simulink model "GaussianDistEstimator"  (R2021b)
settings: Solver=VariableStepAuto  StartTime=0.0  StopTime=10.0  RelTol=1e-3
values from neighbouring files (symbols this model uses):
  nt = 5    [test_disturbance_recursive.m]
  sigma_noise = std_n    (= 0.01)    [test_disturbance_recursive.m]
  tau = [sigma;l]    [test_disturbance_recursive.m]
  tc = 1e-3    (= 0.001)    [test_disturbance_recursive.m]
  v_vbuf = linspace(-1,1,nv)'    [test_disturbance_recursive.m]
libraries: cstblocks x5
settings Model: Creator=manue  LastModifiedBy=manue
settings DataIOCC: ExternalInput=[t, u, v_, n]  LoadExternalInput=on

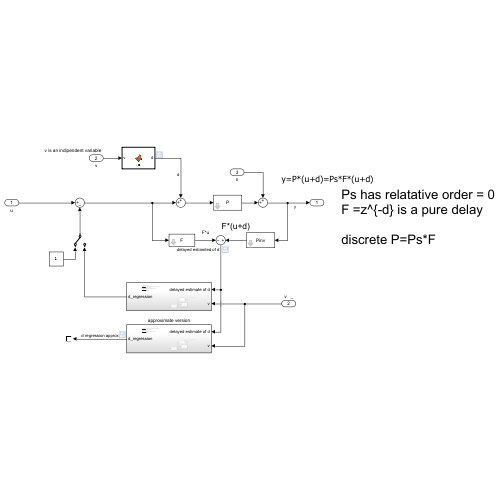
[thumbnail: Simulink's stored preview of the top-level diagram]
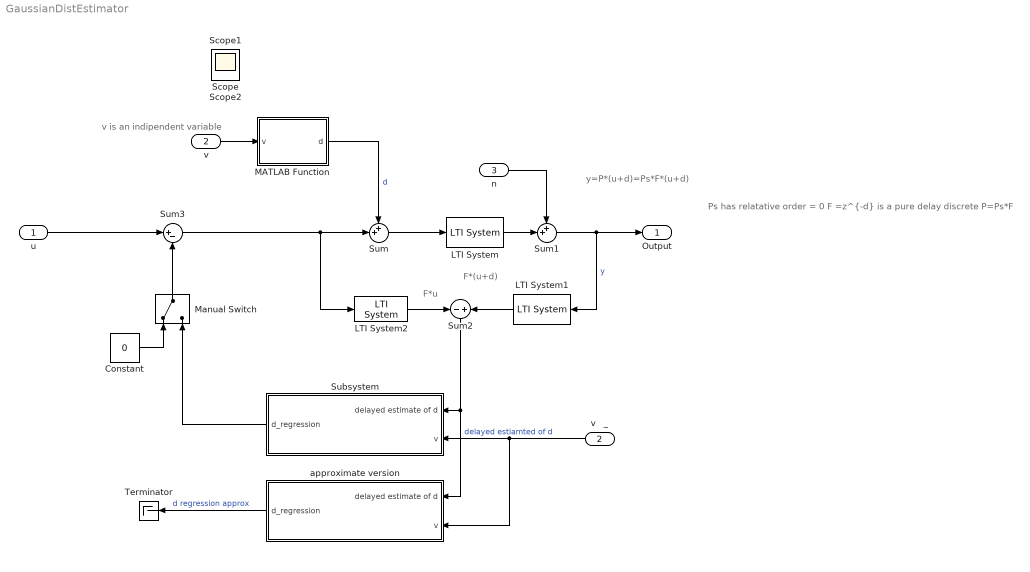
== system GaussianDistEstimator ==
  note: F*u
  note: F*(u+d)
  note: y=P*(u+d)=Ps*F*(u+d)
  note: v is an indipendent variable
  note: Ps has relatative order = 0
      | F =z^{-d} is a pure delay
      |
      | discrete P=Ps*F
  u : Inport
  v : Inport  Port=2
  n : Inport  Port=3
  Constant : Constant  Value=0
  LTI System : cstblocks/LTI System  sys=P  IC=[]
  LTI System1 : cstblocks/LTI System  sys=Pinv  IC=[]
  LTI System2 : cstblocks/LTI System  sys=F  IC=[]
  MATLAB Function : MATLAB Function  TreatAsAtomicUnit=on
  Manual Switch : ManualSwitch
  Subsystem : Subsystem
  Sum : Sum  Inputs=++|
  Sum1 : Sum  Inputs=++|
  Sum2 : Sum  Inputs=-+
  Sum3 : Sum  Inputs=|+-
  Terminator : Terminator
  approximate version : Subsystem
  v   _ : InportShadow  Port=2
  Output : Outport
  Scope : Scope
  Scope1 : Scope
  Scope2 : Scope
  wires:
  Sum/1 -> LTI System/1
  LTI System/1 -> Sum1/2
  Sum3/1 -> LTI System2/1, Sum/2
  Sum1/1 -> LTI System1/1, Output/1  "y"
  v/1 -> MATLAB Function/1(v)
  LTI System2/1 -> Sum2/1
  LTI System1/1 -> Sum2/2
  MATLAB Function/1(d) -> Sum/1  "d"
  u/1 -> Sum3/1
  Manual Switch/1 -> Sum3/2
  Constant/1 -> Manual Switch/1
  n/1 -> Sum1/1
  Sum2/1 -> approximate version/1(delayed estimate of d), Subsystem/1(delayed estimate of d)  "delayed estiamted of d"
  v   _/1 -> approximate version/2(v), Subsystem/2(v)
  Subsystem/1(d_regression) -> Manual Switch/2
  approximate version/1(d_regression) -> Terminator/1  "d regression approx"

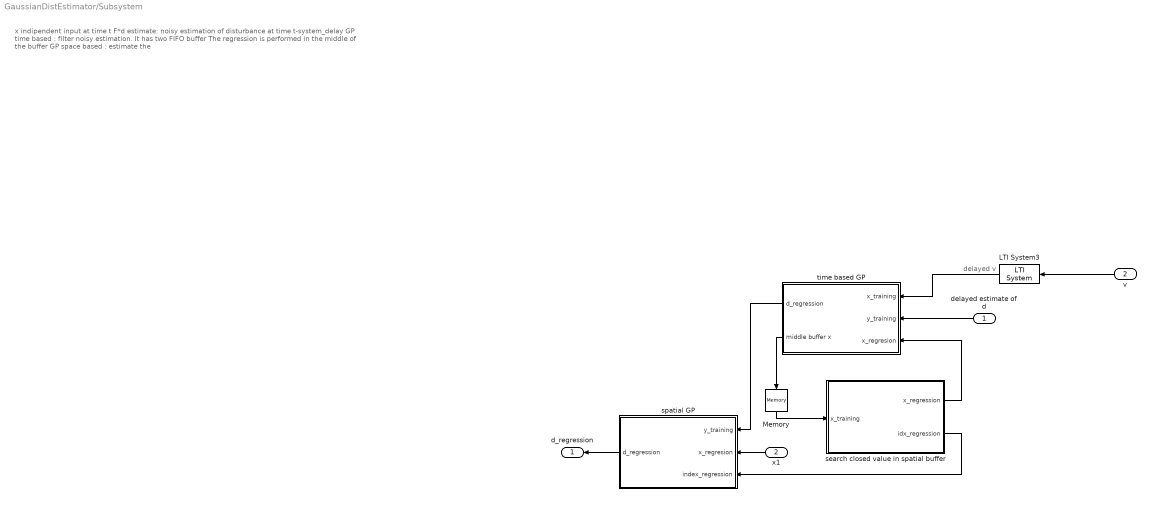
== system GaussianDistEstimator/Subsystem ==
  note: x indipendent input at time t
      | F*d estimate: noisy estimation of disturbance at time t-system_delay
      |
      | GP time based : filter noisy estimation.
      | It has two FIFO buffer
      | The regression is performed in the middle of the buffer
      |
      | GP space based : estimate the
  note: delayed v
  delayed estimate of d : Inport
  v : Inport  Port=2
  LTI System3 : cstblocks/LTI System  sys=F  IC=[]
  Memory : Memory
  search closed value in spatial buffer : Subsystem  TreatAsAtomicUnit=on  SystemSampleTime=tc
  "spatial GP " : Subsystem  TreatAsAtomicUnit=on  SystemSampleTime=tc
  "time based GP " : Subsystem  TreatAsAtomicUnit=on  SystemSampleTime=tc
  x1 : InportShadow  Port=2
  d_regression : Outport
  wires:
  LTI System3/1 -> "time based GP "/1(x_training)
  v/1 -> LTI System3/1
  delayed estimate of d/1 -> "time based GP "/2(y_training)
  "time based GP "/1(d_regression) -> "spatial GP "/1(y_training)
  search closed value in spatial buffer/1(x_regression) -> "time based GP "/3(x_regresion)
  search closed value in spatial buffer/2(idx_regression) -> "spatial GP "/3(index_regression)
  x1/1 -> "spatial GP "/2(x_regresion)
  "spatial GP "/1(d_regression) -> d_regression/1
  "time based GP "/2(middle buffer x) -> Memory/1
  Memory/1 -> search closed value in spatial buffer/1(x_training)

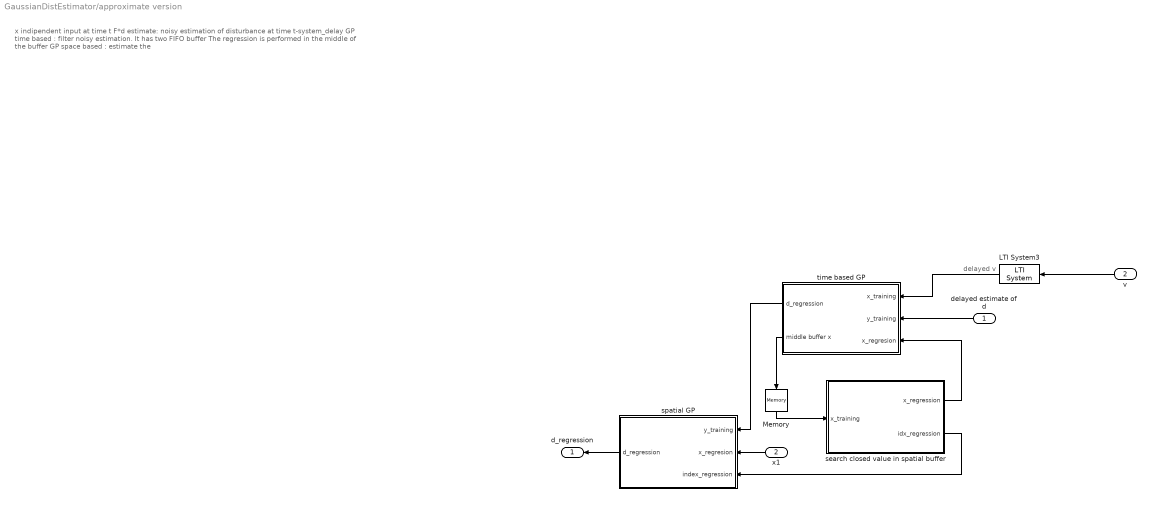
== system GaussianDistEstimator/approximate version ==
  note: delayed v
  note: x indipendent input at time t
      | F*d estimate: noisy estimation of disturbance at time t-system_delay
      |
      | GP time based : filter noisy estimation.
      | It has two FIFO buffer
      | The regression is performed in the middle of the buffer
      |
      | GP space based : estimate the
  delayed estimate of d : Inport
  v : Inport  Port=2
  LTI System3 : cstblocks/LTI System  sys=F  IC=[]
  Memory : Memory
  search closed value in spatial buffer : Subsystem  TreatAsAtomicUnit=on  SystemSampleTime=tc
  "spatial GP " : Subsystem  TreatAsAtomicUnit=on  SystemSampleTime=tc
  "time based GP " : Subsystem  TreatAsAtomicUnit=on  SystemSampleTime=tc
  x1 : InportShadow  Port=2
  d_regression : Outport
  wires:
  Memory/1 -> search closed value in spatial buffer/1(x_training)
  "time based GP "/2(middle buffer x) -> Memory/1
  "spatial GP "/1(d_regression) -> d_regression/1
  x1/1 -> "spatial GP "/2(x_regresion)
  search closed value in spatial buffer/2(idx_regression) -> "spatial GP "/3(index_regression)
  search closed value in spatial buffer/1(x_regression) -> "time based GP "/3(x_regresion)
  "time based GP "/1(d_regression) -> "spatial GP "/1(y_training)
  delayed estimate of d/1 -> "time based GP "/2(y_training)
  v/1 -> LTI System3/1
  LTI System3/1 -> "time based GP "/1(x_training)

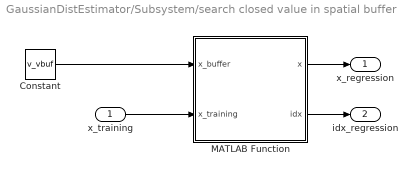
== system GaussianDistEstimator/Subsystem/search closed value in spatial buffer ==
  x_training : Inport
  Constant : Constant  Value=v_vbuf
  MATLAB Function : MATLAB Function  TreatAsAtomicUnit=on
  x_regression : Outport
  idx_regression : Outport  Port=2
  wires:
  Constant/1 -> MATLAB Function/1(x_buffer)
  MATLAB Function/2(idx) -> idx_regression/1
  x_training/1 -> MATLAB Function/2(x_training)
  MATLAB Function/1(x) -> x_regression/1

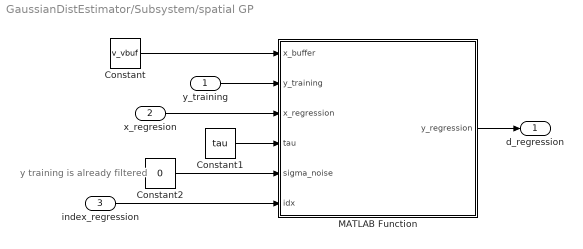
== system GaussianDistEstimator/Subsystem/spatial GP  ==
  note: y training is already filtered
  y_training : Inport
  x_regresion : Inport  Port=2
  index_regression : Inport  Port=3
  Constant : Constant  Value=v_vbuf
  Constant1 : Constant  Value=tau
  Constant2 : Constant  Value=0
  MATLAB Function : MATLAB Function  TreatAsAtomicUnit=on  SystemSampleTime=tc
  d_regression : Outport
  wires:
  MATLAB Function/1(y_regression) -> d_regression/1
  Constant2/1 -> MATLAB Function/5(sigma_noise)
  Constant1/1 -> MATLAB Function/4(tau)
  x_regresion/1 -> MATLAB Function/3(x_regression)
  y_training/1 -> MATLAB Function/2(y_training)
  Constant/1 -> MATLAB Function/1(x_buffer)
  index_regression/1 -> MATLAB Function/6(idx)

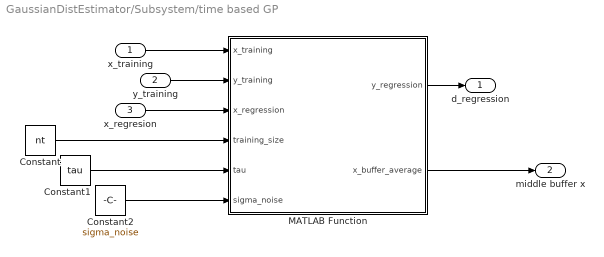
== system GaussianDistEstimator/Subsystem/time based GP  ==
  x_training : Inport
  y_training : Inport  Port=2
  x_regresion : Inport  Port=3
  Constant : Constant  Value=nt
  Constant1 : Constant  Value=tau
  Constant2 : Constant  Value=sigma_noise
  MATLAB Function : MATLAB Function  TreatAsAtomicUnit=on  SystemSampleTime=tc
  d_regression : Outport
  middle buffer x : Outport  Port=2
  wires:
  x_training/1 -> MATLAB Function/1(x_training)
  y_training/1 -> MATLAB Function/2(y_training)
  x_regresion/1 -> MATLAB Function/3(x_regression)
  Constant/1 -> MATLAB Function/4(training_size)
  Constant1/1 -> MATLAB Function/5(tau)
  Constant2/1 -> MATLAB Function/6(sigma_noise)
  MATLAB Function/1(y_regression) -> d_regression/1
  MATLAB Function/2(x_buffer_average) -> middle buffer x/1

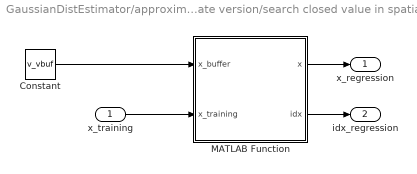
== system GaussianDistEstimator/approximate version/search closed value in spatial buffer ==
  x_training : Inport
  Constant : Constant  Value=v_vbuf
  MATLAB Function : MATLAB Function  TreatAsAtomicUnit=on
  x_regression : Outport
  idx_regression : Outport  Port=2
  wires:
  MATLAB Function/1(x) -> x_regression/1
  x_training/1 -> MATLAB Function/2(x_training)
  MATLAB Function/2(idx) -> idx_regression/1
  Constant/1 -> MATLAB Function/1(x_buffer)

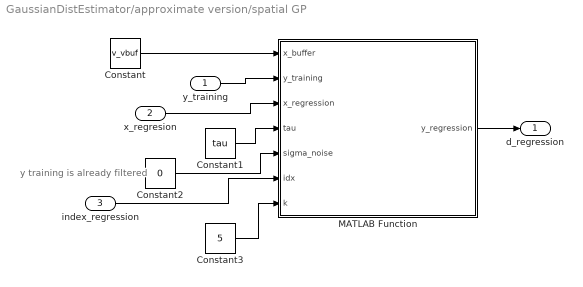
== system GaussianDistEstimator/approximate version/spatial GP  ==
  note: y training is already filtered
  y_training : Inport
  x_regresion : Inport  Port=2
  index_regression : Inport  Port=3
  Constant : Constant  Value=v_vbuf
  Constant1 : Constant  Value=tau
  Constant2 : Constant  Value=0
  Constant3 : Constant  Value=5
  MATLAB Function : MATLAB Function  TreatAsAtomicUnit=on  SystemSampleTime=tc
  d_regression : Outport
  wires:
  index_regression/1 -> MATLAB Function/6(idx)
  Constant/1 -> MATLAB Function/1(x_buffer)
  y_training/1 -> MATLAB Function/2(y_training)
  x_regresion/1 -> MATLAB Function/3(x_regression)
  Constant1/1 -> MATLAB Function/4(tau)
  Constant2/1 -> MATLAB Function/5(sigma_noise)
  MATLAB Function/1(y_regression) -> d_regression/1
  Constant3/1 -> MATLAB Function/7(k)

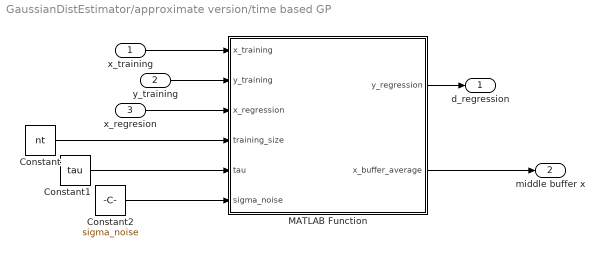
== system GaussianDistEstimator/approximate version/time based GP  ==
  x_training : Inport
  y_training : Inport  Port=2
  x_regresion : Inport  Port=3
  Constant : Constant  Value=nt
  Constant1 : Constant  Value=tau
  Constant2 : Constant  Value=sigma_noise
  MATLAB Function : MATLAB Function  TreatAsAtomicUnit=on  SystemSampleTime=tc
  d_regression : Outport
  middle buffer x : Outport  Port=2
  wires:
  MATLAB Function/2(x_buffer_average) -> middle buffer x/1
  MATLAB Function/1(y_regression) -> d_regression/1
  Constant2/1 -> MATLAB Function/6(sigma_noise)
  Constant1/1 -> MATLAB Function/5(tau)
  Constant/1 -> MATLAB Function/4(training_size)
  x_regresion/1 -> MATLAB Function/3(x_regression)
  y_training/1 -> MATLAB Function/2(y_training)
  x_training/1 -> MATLAB Function/1(x_training)

== matlab function GaussianDistEstimator/Subsystem/spatial GP /MATLAB Function ==
  data: x_buffer input; y_regression output; y_training input; x_regression input; tau input; sigma_noise input; idx input
function y_regression = GP_space_buffer(x_buffer,y_training,x_regression,tau,sigma_noise,idx)

persistent y_buffer kernelFcn K11 pinvK11
if isempty(y_buffer)
    kernelFcn=@(x1,x2)rbf(x1,x2,tau);
    training_size=length(x_buffer);
    y_buffer=zeros(training_size,1);
    K11=kernelFcn(x_buffer,x_buffer)+sigma_noise*eye(training_size);
    pinvK11=pinv(K11);
end

y_buffer(idx)=y_training;
K12=kernelFcn(x_buffer,x_regression);
y_regression=K12'*(pinvK11*y_buffer);

== matlab function GaussianDistEstimator/MATLAB Function ==
  data: v input; d output
function d = fcn(v)

d = 1./(.1+(v-0.5).^2);

== matlab function GaussianDistEstimator/Subsystem/time based GP /MATLAB Function ==
  data: x_training input; y_regression output; y_training input; x_regression input; training_size input; tau input; sigma_noise input; x_buffer_average output
function [y_regression,x_buffer_average] = GP_time_buffer(x_training,y_training,x_regression,training_size,tau,sigma_noise)

persistent x_buffer y_buffer kernelFcn
if isempty(x_buffer)
    kernelFcn=@(x1,x2)rbf(x1,x2,tau);
    x_buffer=zeros(training_size,1);
    y_buffer=zeros(training_size,1);
end

x_buffer=[x_buffer(2:end);x_training];
y_buffer=[y_buffer(2:end);y_training];

K11=kernelFcn(x_buffer,x_buffer)+sigma_noise*eye(training_size);
pinvK11=pinv(K11);

K1a=kernelFcn(x_buffer,x_regression);
y_regression=K1a'*(pinvK11*y_buffer);

x_buffer_average=mean(x_buffer);

== matlab function GaussianDistEstimator/Subsystem/search closed value in spatial buffer/MATLAB Function ==
  data: x output; x_buffer input; idx output; x_training input
function [x,idx] = search_index(x_buffer,x_training)
[a,idx]=min(abs(x_buffer-x_training));
x=x_buffer(idx);

== matlab function GaussianDistEstimator/approximate version/search closed value in spatial buffer/MATLAB Function ==
  data: x output; x_buffer input; idx output; x_training input
function [x,idx] = search_index(x_buffer,x_training)
[a,idx]=min(abs(x_buffer-x_training));
x=x_buffer(idx);

== matlab function GaussianDistEstimator/approximate version/spatial GP /MATLAB Function ==
  data: x_buffer input; y_regression output; y_training input; x_regression input; tau input; sigma_noise input; idx input; k input
function y_regression = GP_space_buffer(x_buffer,y_training,x_regression,tau,sigma_noise,idx,k)

persistent y_buffer kernelFcn 
if isempty(y_buffer)
    kernelFcn=@(x1,x2)rbf(x1,x2,tau);
    training_size=length(x_buffer);
    y_buffer=zeros(training_size,1);
end

y_buffer(idx)=y_training;

[a,idxs]=mink(abs(x_buffer-x_regression),k);

K11=kernelFcn(x_buffer(idxs),x_buffer(idxs))+sigma_noise*eye(k);
pinvK11=pinv(K11);

K12=kernelFcn(x_buffer(idxs),x_regression);
y_regression_=K12'*(pinvK11*y_buffer(idxs));
y_regression=y_regression_(1);% it's already a  scalar, but simulink does not know

== matlab function GaussianDistEstimator/approximate version/time based GP /MATLAB Function ==
  data: x_training input; y_regression output; y_training input; x_regression input; training_size input; tau input; sigma_noise input; x_buffer_average output
function [y_regression,x_buffer_average] = GP_time_buffer(x_training,y_training,x_regression,training_size,tau,sigma_noise)

persistent x_buffer y_buffer kernelFcn
if isempty(x_buffer)
    kernelFcn=@(x1,x2)rbf(x1,x2,tau);
    x_buffer=zeros(training_size,1);
    y_buffer=zeros(training_size,1);
end

x_buffer=[x_buffer(2:end);x_training];
y_buffer=[y_buffer(2:end);y_training];

K11=kernelFcn(x_buffer,x_buffer)+sigma_noise*eye(training_size);
pinvK11=pinv(K11);

K1a=kernelFcn(x_buffer,x_regression);
y_regression=K1a'*(pinvK11*y_buffer);

x_buffer_average=mean(x_buffer);
